simulink model "FTTest07"  (R2013a)
settings: Solver=FixedStepDiscrete  StartTime=0.0  StopTime=inf  FixedStep=0.001  RelTol=1e-3
values from neighbouring files (symbols this model uses):
  MODBUS_TIMEOUT = 0.02    [initFTTest.m]
  STREAMING_TIMEOUT = 0.1    [initFTTest.m]
undefined symbols (not defined in the file or in its folder): FTCalibration, m_XR17D15x, standard
libraries: speedgoatlib x26, xpcseriallib x13, xpclib x1, simulink x1
settings Model: BufferReuse=off  Creator=bgbuss  LastModifiedBy=bgbuss
settings DataIOCC: LimitDataPoints=off
settings OptimizationCC: BlockReduction=off  OptimizeBlockIOStorage=off  BufferReuse=off  ExpressionFolding=off  LocalBlockOutputs=off
settings DebuggingCC: UnderspecifiedInitializationDetection=Simplified
settings HardwareCC: ProdIntDivRoundTo=Zero  ProdEndianess=LittleEndian  ProdHWDeviceType=Generic->32-bit x86 compatible
settings RTWCC: SystemTargetFile=xpctarget.tlc  TemplateMakefile=xpc_default_tmf  Description=xPC Target  ProcessScript=xpctarget_make_rtw_hook  RTWCompilerOptimization=On
settings CodeAppCC: MATLABSourceComments=on
settings xpcTargetCC: TargetFcnLib=ansi_tfl_table_tmw.mat  CodeReplacementLibrary=XPC_BLAS  ParMdlRefBuildCompliant=on  ConcurrentExecutionCompliant=on  CombineSignalStateStructs=off  MATLABClassNameForMDSCustomization=xpcAperiodicCustomization  GRTInterface=on  GenerateAllocFcn=off  RL32LogBufSizeModifier=100000000  xPCTaskExecutionProfile=off  xPCRL32EventNumber=5000  xPCisModelTimeout=off  xPCModelTimeoutSecs=20  xPCLoadParamSetFile=off  xPCConcurrentTasks=off  xPCEnableSFAnimation=off

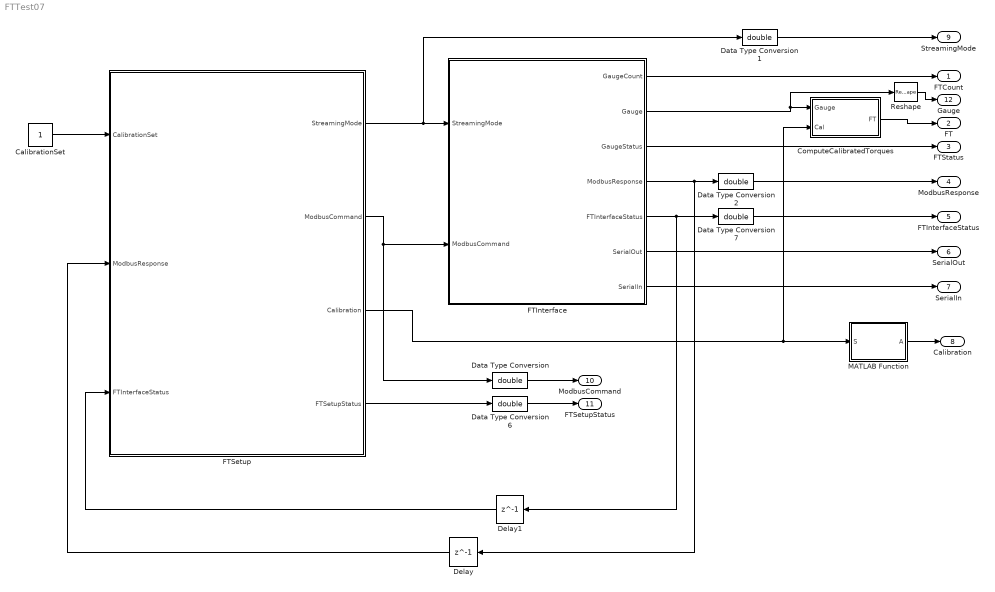
== system FTTest07 ==
  CalibrationSet : Constant
  ComputeCalibratedTorques : Subsystem
  Data Type Conversion{,1..2,6..7} (5 alike) : DataTypeConversion  OutDataTypeStr=double
  Delay : Delay  DelayLength=1  InitialCondition=zeros(256,1,'uint16')
  Delay1 : Delay  DelayLength=1  InitialCondition=0
  FTInterface : Subsystem
  FTSetup : Stateflow chart  TreatAsAtomicUnit=on
  MATLAB Function : MATLAB Function  TreatAsAtomicUnit=on
  Reshape : Reshape
  FTCount : Outport
  FT : Outport  Port=2
  FTStatus : Outport  Port=3
  ModbusResponse : Outport  Port=4
  FTInterfaceStatus : Outport  Port=5
  SerialOut : Outport  Port=6
  SerialIn : Outport  Port=7
  Calibration : Outport  Port=8
  StreamingMode : Outport  Port=9
  ModbusCommand : Outport  Port=10
  FTSetupStatus : Outport  Port=11
  Gauge : Outport  Port=12
  wires:
  FTSetup/1(StreamingMode) -> Data Type Conversion1/1, FTInterface/1(StreamingMode)
  FTInterface/1(GaugeCount) -> FTCount/1
  FTInterface/6(SerialOut) -> SerialOut/1
  FTInterface/7(SerialIn) -> SerialIn/1
  FTSetup/2(ModbusCommand) -> Data Type Conversion/1, FTInterface/2(ModbusCommand)
  FTInterface/4(ModbusResponse) -> Delay/1, Data Type Conversion2/1
  FTInterface/5(FTInterfaceStatus) -> Delay1/1, Data Type Conversion7/1
  CalibrationSet/1 -> FTSetup/1(CalibrationSet)
  FTSetup/3(Calibration) -> MATLAB Function/1(S), ComputeCalibratedTorques/2(Cal)
  MATLAB Function/1(A) -> Calibration/1
  FTInterface/2(Gauge) -> Reshape/1, ComputeCalibratedTorques/1(Gauge)
  Delay/1 -> FTSetup/2(ModbusResponse)
  Delay1/1 -> FTSetup/3(FTInterfaceStatus)
  ComputeCalibratedTorques/1(FT) -> FT/1
  Data Type Conversion/1 -> ModbusCommand/1
  Data Type Conversion1/1 -> StreamingMode/1
  Data Type Conversion2/1 -> ModbusResponse/1
  Data Type Conversion7/1 -> FTInterfaceStatus/1
  Data Type Conversion6/1 -> FTSetupStatus/1
  FTSetup/4(FTSetupStatus) -> Data Type Conversion6/1
  FTInterface/3(GaugeStatus) -> FTStatus/1
  Reshape/1 -> Gauge/1

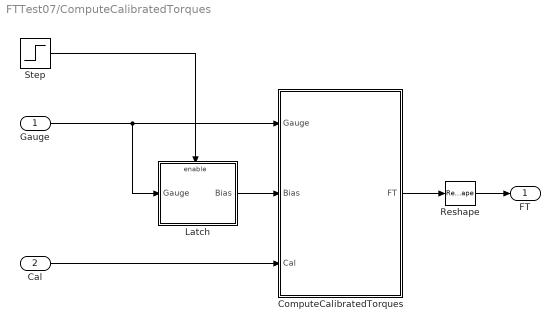
== system FTTest07/ComputeCalibratedTorques ==
  Gauge : Inport
  Cal : Inport  Port=2
  ComputeCalibratedTorques : MATLAB Function  TreatAsAtomicUnit=on
  Latch : Subsystem
  Reshape : Reshape
  Step : Step  Before=1  After=0  SampleTime=0
  FT : Outport
  wires:
  Gauge/1 -> Latch/1(Gauge), ComputeCalibratedTorques/1(Gauge)
  ComputeCalibratedTorques/1(FT) -> Reshape/1
  Cal/1 -> ComputeCalibratedTorques/3(Cal)
  Step/1 -> Latch/Enable
  Latch/1(Bias) -> ComputeCalibratedTorques/2(Bias)
  Reshape/1 -> FT/1

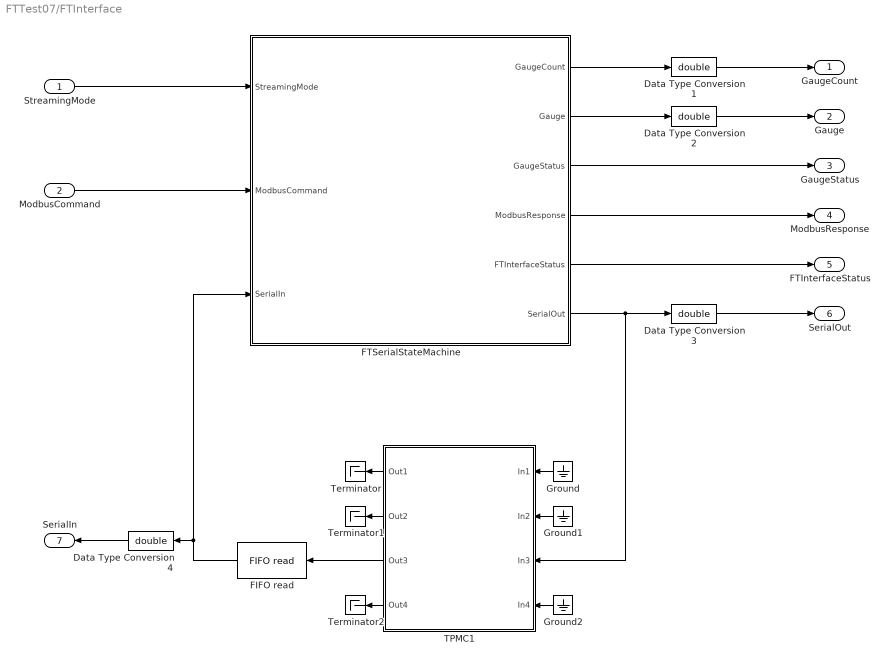
== system FTTest07/FTInterface ==
  StreamingMode : Inport
  ModbusCommand : Inport  Port=2
  Data Type Conversion{1..4} (4 alike) : DataTypeConversion  OutDataTypeStr=double
  "FIFO read " : xpcseriallib/FIFO read   maxsize=255  minsize=1  usedelimiter=off  delimiter=13  outputtype=count+16 bit uint  enable=off  enableout=off  sampletime=0.001
  FTSerialStateMachine : Stateflow chart  TreatAsAtomicUnit=on
  Ground : Ground
  Ground1 : Ground
  Ground2 : Ground
  TPMC1 : Subsystem  AncestorBlock=speedgoatlib/IO503/TPMC466  InitFcn=m_XR17D15x(3);  mask(RS232 Send Receive){group=Basic Setup, port=3, irqnum=5, slot=[4 4], transceiver1=RS485 half-duplex, standard1=on, baud1=115200, bauddivisor1=1, sampling1=16x (standard), prescale1=off, parity1=None, ndata1=8, nstop1=1, rlevel1=1, hwmode1=none, swmode1=none, xonchar1=17, xoffchar1=19, rs485auto1=off, rs485delay1=0, xmtfifosize1=1024, xmtdatatype1=8 bit uint null terminated, rcvfifosize1=1024, transceiver2=RS232 (max 921.6kb/s), standard2=on, baud2=115200, bauddivisor2=1, sampling2=16x (standard), prescale2=off, parity2=None, ndata2=8, nstop2=1, rlevel2=1, hwmode2=none, swmode2=none, xonchar2=17, xoffchar2=19, rs485auto2=off, rs485delay2=0, xmtfifosize2=1024, xmtdatatype2=8 bit uint null terminated, rcvfifosize2=1024, transceiver3=RS485 half-duplex, standard3=on, baud3=1382400, bauddivisor3=1, sampling3=16x (standard), prescale3=off, parity3=Even, ndata3=8, nstop3=1, rlevel3=1, hwmode3=none, swmode3=none, xonchar3=17, xoffchar3=19, rs485auto3=on, rs485delay3=2, xmtfifosize3=128, xmtdatatype3=count+16 bit uint, rcvfifosize3=1024, transceiver4=RS232 (max 921.6kb/s), standard4=on, baud4=115200, bauddivisor4=1, sampling4=16x (standard), prescale4=off, parity4=None, ndata4=8, nstop4=1, rlevel4=half full (32), hwmode4=none, swmode4=none, xonchar4=17, xoffchar4=19, rs485auto4=off, rs485delay4=0, xmtfifosize4=1024, xmtdatatype4=8 bit uint null terminated, rcvfifosize4=1024}
      mask prompts: group "Parameter group:"; port "Port to modify:"; irqnum "IRQ number:"; slot "PCI slot (-1: autosearch):"; transceiver1 "Transceiver setup:"; standard1 "Use standard baud rates (16x, no prescaling)"; baud1 "Standard baud rate:"; bauddivisor1 "Baud rate divisor (non-standard baud rates):"; sampling1 "Sampling rate (non-standard baud rates):"; prescale1 "Prescale by 4 (non-standard baud rates)"; parity1 "Parity:"; ndata1 "Data bits:"; nstop1 "Stop bits:"; rlevel1 "Receive FIFO interrupt level:"; hwmode1 "Hardware handshake:"; swmode1 "Software handshake:"; xonchar1 "XON character:"; xoffchar1 "XOFF character:"; rs485auto1 "RS485 auto turnaround:"; rs485delay1 "RS485 turnaround delay [0,15]"; xmtfifosize1 "Transmit software FIFO size:"; xmtdatatype1 "Transmit FIFO data type:"; rcvfifosize1 "Receive software FIFO size:"; transceiver2 "Transceiver setup:"; standard2 "Use standard baud rates (16x, no prescaling)"; baud2 "Standard baud rate:"; bauddivisor2 "Baud rate divisor (non-standard baud rates):"; sampling2 "Sampling rate (non-standard baud rates):"; prescale2 "Prescale by 4 (non-standard baud rates)"; parity2 "Parity:"; ndata2 "Data bits:"; nstop2 "Stop bits:"; rlevel2 "Receive FIFO interrupt level:"; hwmode2 "Hardware handshake:"; swmode2 "Software handshake:"; xonchar2 "XON character:"; xoffchar2 "XOFF character:"; rs485auto2 "RS485 auto turnaround:"; rs485delay2 "RS485 turnaround delay [0,15]"; xmtfifosize2 "Transmit software FIFO size:"; xmtdatatype2 "Transmit FIFO data type:"; rcvfifosize2 "Receive software FIFO size:"; transceiver3 "Transceiver setup:"; standard3 "Use standard baud rates (16x, no prescaling)"; baud3 "Standard baud rate:"; bauddivisor3 "Baud rate divisor (non-standard baud rates):"; sampling3 "Sampling rate (non-standard baud rates):"; prescale3 "Prescale by 4 (non-standard baud rates)"; parity3 "Parity:"; ndata3 "Data bits:"; nstop3 "Stop bits:"; rlevel3 "Receive FIFO interrupt level:"; hwmode3 "Hardware handshake:"; swmode3 "Software handshake:"; xonchar3 "XON character:"; xoffchar3 "XOFF character:"; rs485auto3 "RS485 auto turnaround:"; rs485delay3 "RS485 turnaround delay [0,15]"; xmtfifosize3 "Transmit software FIFO size:"; xmtdatatype3 "Transmit FIFO data type:"; rcvfifosize3 "Receive software FIFO size:"; transceiver4 "Transceiver setup:"; standard4 "Use standard baud rates (16x, no prescaling)"; baud4 "Standard baud rate:"; bauddivisor4 "Baud rate divisor (non-standard baud rates):"; sampling4 "Sampling rate (non-standard baud rates):"; prescale4 "Prescale by 4 (non-standard baud rates)"; parity4 "Parity:"; ndata4 "Data bits:"; nstop4 "Stop bits:"; rlevel4 "Receive FIFO interrupt level:"; hwmode4 "Hardware handshake:"; swmode4 "Software handshake:"; xonchar4 "XON character:"; xoffchar4 "XOFF character:"; rs485auto4 "RS485 auto turnaround:"; rs485delay4 "RS485 turnaround delay [0,15]"; xmtfifosize4 "Transmit software FIFO size:"; xmtdatatype4 "Transmit FIFO data type:"; rcvfifosize4 "Receive software FIFO size:"
      mask help:
      | PMC521
      | Acromag
      | EIA/TIA-422B Send Receive Subsystem
      mask init:
      | brdslot = slot;
      | m_tews_XR17D15x(1, 4);
      mask Help: helpview(fullfile(docroot, 'mapfiles', 'xpc.map'), 'Commtech_Subsystem')
      mask TypeOptions group: Board Setup | Basic Setup | FIFO Setup
      mask Callback group: m_tews_XR17D15x(2, 4);
      mask TypeOptions port: 1 | 2 | 3 | 4
      mask Callback port: m_tews_XR17D15x(2, 4);
      mask TypeOptions transceiver1: RS232 (max 921.6kb/s) | RS422 | RS422 multidrop | RS485 full-duplex | RS485 half-duplex
      mask TypeOptions baud1: 2764800 | 1382400 | 921600 | 460800 | 230400 | 115200 | 57600 | 38400 | 19200 | 9600 | 4800 | 2400 | 1200 | 600 | 400
      mask TypeOptions sampling1: 8x | 16x (standard)
      mask TypeOptions parity1: None | Even | Odd | Mark | Space
      mask TypeOptions ndata1: 5 | 6 | 7 | 8
      mask TypeOptions nstop1: 1 | 2
      mask TypeOptions rlevel1: 1 | quarter full (16) | half full (32) | almost full (56)
      mask TypeOptions hwmode1: RTS/CTS | none
      mask TypeOptions swmode1: XON/XOFF | none
      mask TypeOptions xmtdatatype1: count+32 bit int | count+32 bit uint | count+16 bit int | count+16 bit uint | 8 bit int null terminated | 8 bit uint null terminated
      mask TypeOptions transceiver2: RS232 (max 921.6kb/s) | RS422 | RS422 multidrop | RS485 full-duplex | RS485 half-duplex
      mask TypeOptions baud2: 2764800 | 1382400 | 921600 | 460800 | 230400 | 115200 | 57600 | 38400 | 19200 | 9600 | 4800 | 2400 | 1200 | 600 | 400
      mask TypeOptions sampling2: 8x | 16x (standard)
      mask TypeOptions parity2: None | Even | Odd | Mark | Space
      mask TypeOptions ndata2: 5 | 6 | 7 | 8
      mask TypeOptions nstop2: 1 | 2
      mask TypeOptions rlevel2: 1 | quarter full (16) | half full (32) | almost full (56)
      mask TypeOptions hwmode2: RTS/CTS | none
      mask TypeOptions swmode2: XON/XOFF | none
      mask TypeOptions xmtdatatype2: count+32 bit int | count+32 bit uint | count+16 bit int | count+16 bit uint | 8 bit int null terminated | 8 bit uint null terminated
      mask TypeOptions transceiver3: RS232 (max 921.6kb/s) | RS422 | RS422 multidrop | RS485 full-duplex | RS485 half-duplex
      mask TypeOptions baud3: 2764800 | 1382400 | 921600 | 460800 | 230400 | 115200 | 57600 | 38400 | 19200 | 9600 | 4800 | 2400 | 1200 | 600 | 400
      mask TypeOptions sampling3: 8x | 16x (standard)
      mask TypeOptions parity3: None | Even | Odd | Mark | Space
      mask TypeOptions ndata3: 5 | 6 | 7 | 8
      mask TypeOptions nstop3: 1 | 2
      mask TypeOptions rlevel3: 1 | quarter full (16) | half full (32) | almost full (56)
      mask TypeOptions hwmode3: RTS/CTS | none
      mask TypeOptions swmode3: XON/XOFF | none
      mask TypeOptions xmtdatatype3: count+32 bit int | count+32 bit uint | count+16 bit int | count+16 bit uint | 8 bit int null terminated | 8 bit uint null terminated
      mask TypeOptions transceiver4: RS232 (max 921.6kb/s) | RS422 | RS422 multidrop | RS485 full-duplex | RS485 half-duplex
      mask TypeOptions baud4: 2764800 | 1382400 | 921600 | 460800 | 230400 | 115200 | 57600 | 38400 | 19200 | 9600 | 4800 | 2400 | 1200 | 600 | 400
      mask TypeOptions sampling4: 8x | 16x (standard)
      mask TypeOptions parity4: None | Even | Odd | Mark | Space
      mask TypeOptions ndata4: 5 | 6 | 7 | 8
      mask TypeOptions nstop4: 1 | 2
      mask TypeOptions rlevel4: 1 | quarter full (16) | half full (32) | almost full (56)
      mask TypeOptions hwmode4: RTS/CTS | none
      mask TypeOptions swmode4: XON/XOFF | none
      mask TypeOptions xmtdatatype4: count+32 bit int | count+32 bit uint | count+16 bit int | count+16 bit uint | 8 bit int null terminated | 8 bit uint null terminated
      mask Display:
      | disp('TEWS\nTPMC466\nRS232/422/485\nSend\nReceive');
      | port_label( 'input', 1, 'XMT1' );
      | port_label( 'input', 2, 'XMT2' );
      | port_label( 'input', 3, 'XMT3' );
      | port_label( 'input', 4, 'XMT4' );
      | 
      | port_label( 'output', 1, 'FIFO1' );
      | port_label( 'output', 2, 'FIFO2' );
      | port_label( 'output', 3, 'FIFO3' );
      | port_label( 'output', 4, 'FIFO4' );
  Terminator : Terminator
  Terminator1 : Terminator
  Terminator2 : Terminator
  GaugeCount : Outport
  Gauge : Outport  Port=2
  GaugeStatus : Outport  Port=3
  ModbusResponse : Outport  Port=4
  FTInterfaceStatus : Outport  Port=5
  SerialOut : Outport  Port=6
  SerialIn : Outport  Port=7
  wires:
  FTSerialStateMachine/2(Gauge) -> Data Type Conversion2/1
  Data Type Conversion2/1 -> Gauge/1
  FTSerialStateMachine/1(GaugeCount) -> Data Type Conversion1/1
  TPMC1/3(Out3) -> "FIFO read "/1
  ModbusCommand/1 -> FTSerialStateMachine/2(ModbusCommand)
  TPMC1/1(Out1) -> Terminator/1
  TPMC1/2(Out2) -> Terminator1/1
  TPMC1/4(Out4) -> Terminator2/1
  Ground/1 -> TPMC1/1(In1)
  Ground2/1 -> TPMC1/4(In4)
  Ground1/1 -> TPMC1/2(In2)
  FTSerialStateMachine/4(ModbusResponse) -> ModbusResponse/1
  Data Type Conversion1/1 -> GaugeCount/1
  Data Type Conversion3/1 -> SerialOut/1
  "FIFO read "/1 -> Data Type Conversion4/1, FTSerialStateMachine/3(SerialIn)
  Data Type Conversion4/1 -> SerialIn/1
  StreamingMode/1 -> FTSerialStateMachine/1(StreamingMode)
  FTSerialStateMachine/5(FTInterfaceStatus) -> FTInterfaceStatus/1
  FTSerialStateMachine/6(SerialOut) -> Data Type Conversion3/1, TPMC1/3(In3)
  FTSerialStateMachine/3(GaugeStatus) -> GaugeStatus/1

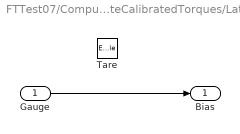
== system FTTest07/ComputeCalibratedTorques/Latch ==
  Gauge : Inport
  Tare : EnablePort
  Bias : Outport  InitialOutput=zeros(6,8,'uint16')
  wires:
  Gauge/1 -> Bias/1

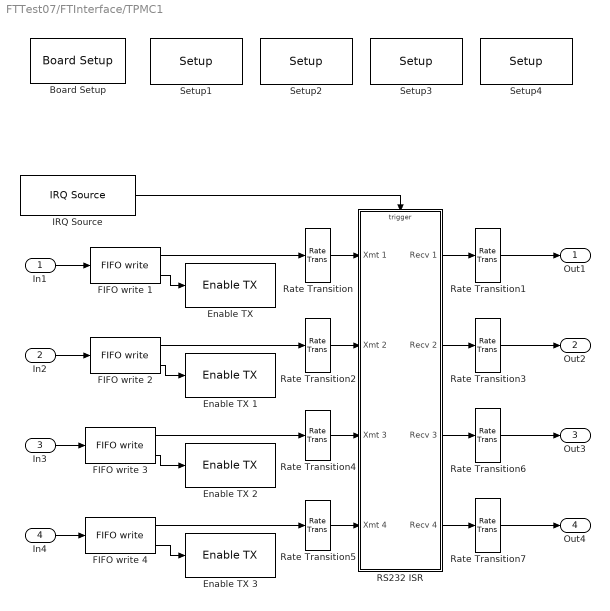
== system FTTest07/FTInterface/TPMC1 ==
  In1 : Inport
  In2 : Inport  Port=2
  In3 : Inport  Port=3
  In4 : Inport  Port=4
  Board Setup : speedgoatlib/IO503/TEWS TPMC466 Internal blocks/Board Setup  irqnum=5  slot=brdslot
  "Enable TX " : speedgoatlib/IO503/TEWS TPMC466 Internal blocks/Enable TX   port=1  slot=brdslot
  Enable TX 1 : speedgoatlib/IO503/TEWS TPMC466 Internal blocks/Enable TX   port=2  slot=brdslot
  Enable TX 2 : speedgoatlib/IO503/TEWS TPMC466 Internal blocks/Enable TX   port=3  slot=brdslot
  Enable TX 3 : speedgoatlib/IO503/TEWS TPMC466 Internal blocks/Enable TX   port=4  slot=brdslot
  FIFO write 1 : xpcseriallib/FIFO write   size=1024  inputtype=8 bit uint null terminated  present=on  sampletime=-1  id=XMT channel 1, IRQ 5
  FIFO write 2 : xpcseriallib/FIFO write   size=1024  inputtype=8 bit uint null terminated  present=on  sampletime=-1  id=XMT channel 2, IRQ 5
  FIFO write 3 : xpcseriallib/FIFO write   size=128  inputtype=count+16 bit uint  present=on  sampletime=-1  id=XMT channel 3, IRQ 5
  FIFO write 4 : xpcseriallib/FIFO write   size=1024  inputtype=8 bit uint null terminated  present=on  sampletime=-1  id=XMT channel 4, IRQ 5
  IRQ Source : xpclib/Asynchronous Event/IRQ Source  irqNo=5  preempt=off  b_type=None/Other  slot=brdslot
  RS232 ISR : Subsystem  TreatAsAtomicUnit=on  mask(RS232 ISR){slot=brdslot}
      mask help:
      | PMC521
      | Acromag
      | Interrupt Service Routine
      mask init:
      | subslot = slot;
      mask Display:
      | disp('PMC521\nAcromag\nISR');
      | port_label('input', 1, 'XMT1');
      | port_label('input', 2, 'XMT2');
      | port_label('input', 3, 'XMT3');
      | port_label('input', 4, 'XMT4');
      | port_label('input', 5, 'XMT5');
      | port_label('input', 6, 'XMT6');
      | port_label('input', 7, 'XMT7');
      | port_label('input', 8, 'XMT8');
      | port_label('output', 1, 'RCV1');
      | port_label('output', 2, 'RCV2');
      | port_label('output', 3, 'RCV3');
      | port_label('output', 4, 'RCV4');
      | port_label('output', 5, 'RCV5');
      | port_label('output', 6, 'RCV6');
      | port_label('output', 7, 'RCV7');
      | port_label('output', 8, 'RCV8');
  Rate Transition{,2,4..5} (4 alike) : RateTransition  Integrity=off  Deterministic=off
  Rate Transition{1,3,6..7} (4 alike) : RateTransition  Integrity=off  Deterministic=off  OutPortSampleTime=0
  Setup1 : speedgoatlib/IO503/TEWS TPMC466 Internal blocks/Setup   port=1  transceiver=RS485 half-duplex  standard=on  baudrate=115200  bauddivisor=1  mode8x=16x (standard)  prescale=off  width=8  nstop=1  parity=None  rlevel=1  ctsmode=none  xonoff=none  xon=17  xoff=19  rs485mode=off  rs485delay=0  slot=brdslot
  Setup2 : speedgoatlib/IO503/TEWS TPMC466 Internal blocks/Setup   port=2  transceiver=RS232 (max 921.6kb/s)  standard=on  baudrate=115200  bauddivisor=1  mode8x=16x (standard)  prescale=off  width=8  nstop=1  parity=None  rlevel=1  ctsmode=none  xonoff=none  xon=17  xoff=19  rs485mode=off  rs485delay=0  slot=brdslot
  Setup3 : speedgoatlib/IO503/TEWS TPMC466 Internal blocks/Setup   port=3  transceiver=RS485 half-duplex  standard=on  baudrate=1382400  bauddivisor=1  mode8x=16x (standard)  prescale=off  width=8  nstop=1  parity=Even  rlevel=1  ctsmode=none  xonoff=none  xon=17  xoff=19  rs485mode=on  rs485delay=2  slot=brdslot
  Setup4 : speedgoatlib/IO503/TEWS TPMC466 Internal blocks/Setup   port=4  transceiver=RS232 (max 921.6kb/s)  standard=on  baudrate=115200  bauddivisor=1  mode8x=16x (standard)  prescale=off  width=8  nstop=1  parity=None  rlevel=half full (32)  ctsmode=none  xonoff=none  xon=17  xoff=19  rs485mode=off  rs485delay=0  slot=brdslot
  Out1 : Outport
  Out2 : Outport  Port=2
  Out3 : Outport  Port=3
  Out4 : Outport  Port=4
  wires:
  RS232 ISR/4(Recv 4) -> Rate Transition7/1
  RS232 ISR/3(Recv 3) -> Rate Transition6/1
  Rate Transition7/1 -> Out4/1
  Rate Transition6/1 -> Out3/1
  Rate Transition5/1 -> RS232 ISR/4(Xmt 4)
  Rate Transition4/1 -> RS232 ISR/3(Xmt 3)
  FIFO write 4/1 -> Rate Transition5/1
  In4/1 -> FIFO write 4/1
  FIFO write 4/2 -> Enable TX 3/1
  FIFO write 3/1 -> Rate Transition4/1
  In3/1 -> FIFO write 3/1
  FIFO write 3/2 -> Enable TX 2/1
  Rate Transition1/1 -> Out1/1
  Rate Transition3/1 -> Out2/1
  Rate Transition/1 -> RS232 ISR/1(Xmt 1)
  Rate Transition2/1 -> RS232 ISR/2(Xmt 2)
  FIFO write 1/2 -> "Enable TX "/1
  IRQ Source/1 -> RS232 ISR/Trigger
  RS232 ISR/1(Recv 1) -> Rate Transition1/1
  RS232 ISR/2(Recv 2) -> Rate Transition3/1
  FIFO write 1/1 -> Rate Transition/1
  In1/1 -> FIFO write 1/1
  FIFO write 2/1 -> Rate Transition2/1
  In2/1 -> FIFO write 2/1
  FIFO write 2/2 -> Enable TX 1/1

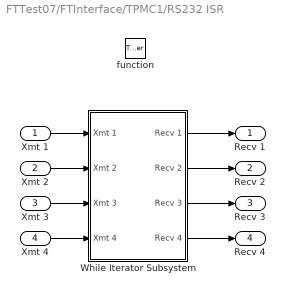
== system FTTest07/FTInterface/TPMC1/RS232 ISR ==
  Xmt 1 : Inport
  Xmt 2 : Inport  Port=2
  Xmt 3 : Inport  Port=3
  Xmt 4 : Inport  Port=4
  function : TriggerPort  TriggerType=function-call
  While Iterator Subsystem : Subsystem  TreatAsAtomicUnit=on
  Recv 1 : Outport  SourceOfInitialOutputValue=Input signal
  Recv 2 : Outport  Port=2  SourceOfInitialOutputValue=Input signal
  Recv 3 : Outport  Port=3  SourceOfInitialOutputValue=Input signal
  Recv 4 : Outport  Port=4  SourceOfInitialOutputValue=Input signal
  wires:
  While Iterator Subsystem/4(Recv 4) -> Recv 4/1
  While Iterator Subsystem/3(Recv 3) -> Recv 3/1
  Xmt 4/1 -> While Iterator Subsystem/4(Xmt 4)
  Xmt 3/1 -> While Iterator Subsystem/3(Xmt 3)
  While Iterator Subsystem/2(Recv 2) -> Recv 2/1
  While Iterator Subsystem/1(Recv 1) -> Recv 1/1
  Xmt 2/1 -> While Iterator Subsystem/2(Xmt 2)
  Xmt 1/1 -> While Iterator Subsystem/1(Xmt 1)

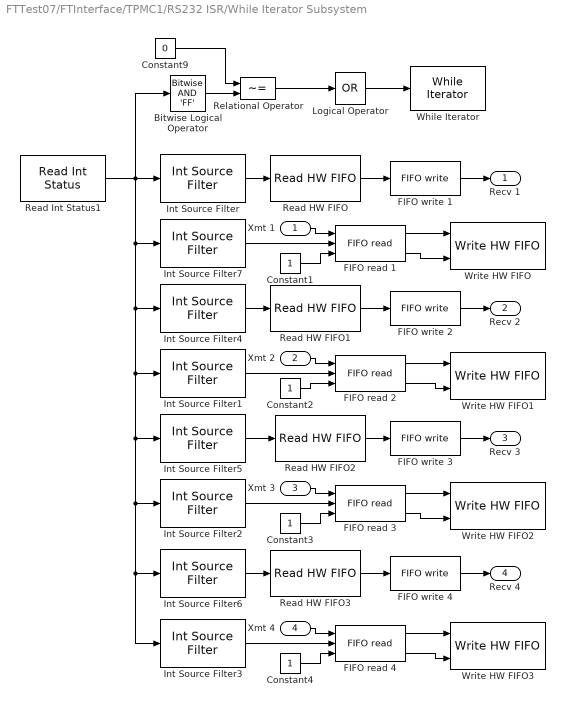
== system FTTest07/FTInterface/TPMC1/RS232 ISR/While Iterator Subsystem ==
  Xmt 1 : Inport
  Xmt 2 : Inport  Port=2
  Xmt 3 : Inport  Port=3
  Xmt 4 : Inport  Port=4
  Bitwise Logical Operator : simulink/Logic and Bit Operations/Bitwise Operator  logicop=AND  UseBitMask=on  BitMask='FF'  BitMaskRealWorld=Stored Integer
  Constant{1..4} (4 alike) : Constant  OutDataTypeStr=uint32
  Constant9 : Constant  Value=0  OutDataTypeStr=uint32
  FIFO read {1..4} (4 alike) : xpcseriallib/FIFO read   maxsize=60  minsize=1  usedelimiter=off  delimiter=13  outputtype=count+32 bit uint  enable=on  enableout=on  sampletime=-1
  FIFO write 1 : xpcseriallib/FIFO write   size=1024  inputtype=count+32 bit uint  present=off  sampletime=-1  id=RCV channel 1, IRQ 5
  FIFO write 2 : xpcseriallib/FIFO write   size=1024  inputtype=count+32 bit uint  present=off  sampletime=-1  id=RCV channel 2, IRQ 5
  FIFO write 3 : xpcseriallib/FIFO write   size=1024  inputtype=count+32 bit uint  present=off  sampletime=-1  id=RCV channel 3, IRQ 5
  FIFO write 4 : xpcseriallib/FIFO write   size=1024  inputtype=count+32 bit uint  present=off  sampletime=-1  id=RCV channel 4, IRQ 5
  Int Source Filter : speedgoatlib/IO503/TEWS TPMC466 Internal blocks/Int Source Filter  port=1  value=Receive data
  Int Source Filter1 : speedgoatlib/IO503/TEWS TPMC466 Internal blocks/Int Source Filter  port=2  value=Transmitter empty
  Int Source Filter2 : speedgoatlib/IO503/TEWS TPMC466 Internal blocks/Int Source Filter  port=3  value=Transmitter empty
  Int Source Filter3 : speedgoatlib/IO503/TEWS TPMC466 Internal blocks/Int Source Filter  port=4  value=Transmitter empty
  Int Source Filter4 : speedgoatlib/IO503/TEWS TPMC466 Internal blocks/Int Source Filter  port=2  value=Receive data
  Int Source Filter5 : speedgoatlib/IO503/TEWS TPMC466 Internal blocks/Int Source Filter  port=3  value=Receive data
  Int Source Filter6 : speedgoatlib/IO503/TEWS TPMC466 Internal blocks/Int Source Filter  port=4  value=Receive data
  Int Source Filter7 : speedgoatlib/IO503/TEWS TPMC466 Internal blocks/Int Source Filter  port=1  value=Transmitter empty
  Logical Operator : Logic  Operator=OR  Inputs=1  AllPortsSameDT=off
  Read HW FIFO : speedgoatlib/IO503/TEWS TPMC466 Internal blocks/Read HW FIFO  port=1  flush=on  slot=subslot
  Read HW FIFO1 : speedgoatlib/IO503/TEWS TPMC466 Internal blocks/Read HW FIFO  port=2  flush=on  slot=subslot
  Read HW FIFO2 : speedgoatlib/IO503/TEWS TPMC466 Internal blocks/Read HW FIFO  port=3  flush=on  slot=subslot
  Read HW FIFO3 : speedgoatlib/IO503/TEWS TPMC466 Internal blocks/Read HW FIFO  port=4  flush=on  slot=subslot
  Read Int Status1 : speedgoatlib/IO503/TEWS TPMC466 Internal blocks/Read Int Status  slot=subslot
  Relational Operator : RelationalOperator  Operator=~=
  While Iterator : WhileIterator  MaxIters=65  WhileBlockType=do-while
  Write HW FIFO : speedgoatlib/IO503/TEWS TPMC466 Internal blocks/Write HW FIFO  port=1  slot=subslot
  Write HW FIFO1 : speedgoatlib/IO503/TEWS TPMC466 Internal blocks/Write HW FIFO  port=2  slot=subslot
  Write HW FIFO2 : speedgoatlib/IO503/TEWS TPMC466 Internal blocks/Write HW FIFO  port=3  slot=subslot
  Write HW FIFO3 : speedgoatlib/IO503/TEWS TPMC466 Internal blocks/Write HW FIFO  port=4  slot=subslot
  Recv 1 : Outport  SourceOfInitialOutputValue=Input signal
  Recv 2 : Outport  Port=2  SourceOfInitialOutputValue=Input signal
  Recv 3 : Outport  Port=3  SourceOfInitialOutputValue=Input signal
  Recv 4 : Outport  Port=4  SourceOfInitialOutputValue=Input signal
  wires:
  Read HW FIFO3/1 -> FIFO write 4/1
  FIFO write 4/1 -> Recv 4/1
  Read HW FIFO2/1 -> FIFO write 3/1
  FIFO write 3/1 -> Recv 3/1
  Int Source Filter6/1 -> Read HW FIFO3/1
  Int Source Filter5/1 -> Read HW FIFO2/1
  Constant3/1 -> FIFO read 3/3
  FIFO read 3/2 -> Write HW FIFO2/2
  FIFO read 3/1 -> Write HW FIFO2/1
  Xmt 3/1 -> FIFO read 3/1
  Int Source Filter2/1 -> FIFO read 3/2
  Constant2/1 -> FIFO read 2/3
  Constant1/1 -> FIFO read 1/3
  FIFO read 2/2 -> Write HW FIFO1/2
  FIFO read 1/2 -> Write HW FIFO/2
  FIFO read 1/1 -> Write HW FIFO/1
  FIFO read 2/1 -> Write HW FIFO1/1
  Xmt 2/1 -> FIFO read 2/1
  Int Source Filter1/1 -> FIFO read 2/2
  Read HW FIFO1/1 -> FIFO write 2/1
  FIFO write 2/1 -> Recv 2/1
  Int Source Filter4/1 -> Read HW FIFO1/1
  Xmt 1/1 -> FIFO read 1/1
  Int Source Filter7/1 -> FIFO read 1/2
  Read HW FIFO/1 -> FIFO write 1/1
  FIFO write 1/1 -> Recv 1/1
  Int Source Filter/1 -> Read HW FIFO/1
  Read Int Status1/1 -> Bitwise Logical Operator/1, Int Source Filter6/1, Int Source Filter3/1, Int Source Filter2/1, Int Source Filter5/1, Int Source Filter1/1, Int Source Filter4/1, Int Source Filter7/1, Int Source Filter/1
  Constant9/1 -> Relational Operator/1
  Bitwise Logical Operator/1 -> Relational Operator/2
  Relational Operator/1 -> Logical Operator/1
  Logical Operator/1 -> While Iterator/1
  Constant4/1 -> FIFO read 4/3
  FIFO read 4/2 -> Write HW FIFO3/2
  FIFO read 4/1 -> Write HW FIFO3/1
  Xmt 4/1 -> FIFO read 4/1
  Int Source Filter3/1 -> FIFO read 4/2

== stateflow chart FTTest07/FTSetup ==
  state Initialize
    entry:
    FTSetupStatus = 0;
    clearModbusCommand();
    clearCalibration();
    StreamingMode = 0;
  state ModbusMode
    entry:
    FTSetupStatus = 1;
    clearModbusCommand();
    clearCalibration();
    StreamingMode = 0;
    state SetSessionId
      entry:
      FTSetupStatus = 1.10;
    state ReadCalibration
      entry:
      FTSetupStatus = 1.20;
      state SendRequest1
        entry:
        FTSetupStatus = 1.21;
        requestCalibration(1);
        during:
        clearModbusCommand();
      state SendRequest2
        entry:
        FTSetupStatus = 1.23;
        requestCalibration(2);
        during:
        clearModbusCommand();
      state ParseRequest1
        entry:
        FTSetupStatus = 1.22;
        parseCalibration(1);
      state ParseRequest2
        entry:
        FTSetupStatus = 1.24;
        parseCalibration(2);
      (default) -> SendRequest1
      SendRequest1 -> SendRequest1 [order 2] : [after(0.2,sec)]
      SendRequest2 -> SendRequest2 [order 2] : [after(0.2, sec)]
      ParseRequest1 -> SendRequest2
      SendRequest1 -> ParseRequest1 [order 1] : [validResponse()]
      SendRequest2 -> ParseRequest2 [order 1] : [validResponse()]
    state WriteActiveCalibration
      entry:
      FTSetupStatus = 1.30;
      (history)
      state LockStorage
        entry:
        FTSetupStatus = 1.34;
        lockUnlockStorage(0);
        during:
        clearModbusCommand();
      state writeActiveCal
        entry:
        FTSetupStatus = 1.33;
        writeActiveCalibration();
        during:
        clearModbusCommand();
      state readActiveCal
        entry:
        FTSetupStatus = 1.31;
        readActiveCalibration();
        during:
        clearModbusCommand();
      state UnlockStorage
        entry:
        FTSetupStatus = 1.32;
        lockUnlockStorage(1);
        during:
        clearModbusCommand();
      (default) -> readActiveCal
      writeActiveCal -> LockStorage : [validResponse()]
      LockStorage -> readActiveCal : [validResponse()]
      UnlockStorage -> writeActiveCal : [validResponse()]
      readActiveCal -> UnlockStorage [order 2] : [validResponse()]
    (default) -> SetSessionId
    SetSessionId -> ReadCalibration
    ParseRequest2 -> WriteActiveCalibration
    WriteActiveCalibration -> WriteActiveCalibration : [after(2*MODBUS_TIMEOUT, sec)]
  state StreamingMode
    entry:
    FTSetupStatus = 2;
    clearModbusCommand();
    StreamingMode = 1;
  (default) -> Initialize
  Initialize -> ModbusMode : [abs(FTInterfaceStatus - 1.1) < 0.0001]
  readActiveCal -> StreamingMode [order 1] : [validResponse() && verifyActiveCalibration()]
  data: valid function_output; Part function_input; Part function_input; ok function_output; Unlock function_input; CalibrationSet input; StreamingMode output; ModbusResponse input; FTInterfaceStatus input; ModbusCommand output uint16 size=256; Calibration output Bus: FTCalibrationBus; FTCalibration parameter Bus: FTCalibrationBus; FTSetupStatus output; CalibrationBuffer local; CalibrationBufferEnd local; MODBUS_TIMEOUT parameter
  function clearModbusCommand:
    | function clearModbusCommand %#codegen
    |     ModbusCommand = zeros(256,1,'uint16');
    | end
  function clearCalibration:
    | function clearCalibration %#codegen
    |     Calibration       = FTCalibration;
    |     CalibrationBuffer = zeros(512,1,'uint16');
    |     CalibrationBufferEnd = uint16(0);
    | end
  function valid = validResponse:
    | function valid = validResponse %#codegen
    |     valid = false;
    |     
    |     if (ModbusResponse(1) > 1)    
    |         switch (ModbusResponse(2))
    |             case uint16(3)
    |                 valid = true;
    |             case uint16(6)
    |                 valid = true;
    |             case uint16(16)
    |                 valid = true;
    |             case uint16(70)
    |                 valid = (ModbusResponse(3) == uint16(1));
    |             case uint16(106)
    |                 valid = (ModbusResponse(3) == uint16(1));
    |         end
    |     end
    | end
  function requestCalibration(Part):
    | function requestCalibration(Part) %#codegen
    |    % ATI F/T Calibration data are stored in holding registers. There are 16
    |    % calibration sets, each 338 bytes (or 169 16-bit holding registers)
    |    % long. They are stored beginning at holding register address 0x00e3
    |    % (Calibration 1) 192 holding registers apart.
    |    Address = uint16(hex2dec('00e3')) + uint16(192 * (CalibrationSet - 1));
    |    
    |    % Calibration data must be read in two or more parts due to length
    |    % restricitons in the Modbus protocol.
    |    NumRegs1 = 85;
    |    NumRegs2 = 84;
    |    if (Part==1)
    |        NumRegs = NumRegs1;
    |    else
    |        NumRegs = NumRegs2;
    |        Address = Address + uint16(NumRegs1);
    |    end
    |    ModbusFunction = 3;
    |    ModbusCommand(1:6) = uint16([5; ModbusFunction; bitshift(Address,-8); bitand(Address,255); 0; NumRegs]);
    | end
  function parseCalibration(Part):
    | function parseCalibration(Part) %#codegen
    |     % Calibration data must be read in two or more parts due to length
    |     % restricitons in the Modbus protocol.
    |     if (Part==1)
    |         CalibrationBuffer(1:ModbusResponse(3)) = ModbusResponse(3+(1:ModbusResponse(3)));
    |         CalibrationBufferEnd = ModbusResponse(3);
    |     else
    |         CalibrationBuffer(CalibrationBufferEnd+(1:ModbusResponse(3))) = ModbusResponse(3+(1:ModbusResponse(3)));
    |         CalibrationBufferEndTemp = CalibrationBufferEnd + ModbusResponse(3);
    |         Calibration = parseFTCalibration2(CalibrationBuffer(1:CalibrationBufferEndTemp));
    |     end
    | end
    | 
    | function Cal = parseFTCalibration2(CalibrationBuffer)
    |     Cal.CalibSerialNumber = parseUint8(CalibrationBuffer(1:8));
    |     Cal.CalibPartNumber   = parseUint8(CalibrationBuffer(9:40));
    |     Cal.CalibFamilyId     = parseUint8(CalibrationBuffer(41:44));
    |     Cal.CalibTime         = parseUint8(CalibrationBuffer(45:64));
    |     Cal.BasicMatrix       = reshape(parseFloat(CalibrationBuffer(65:208)), 6, 6).';
    |     Cal.ForceUnits        = parseUint8(CalibrationBuffer(209));
    |     Cal.TorqueUnits       = parseUint8(CalibrationBuffer(210));
    |     Cal.MaxRating         = parseFloat(CalibrationBuffer(211:234));
    |     Cal.CountsPerForce    = parseInt32(CalibrationBuffer(235:238));
    |     Cal.CountsPerTorque   = parseInt32(CalibrationBuffer(239:242));
    |     Cal.GageGain          = parseUint16(CalibrationBuffer(243:254));
    |     Cal.GageOffset        = parseUint16(CalibrationBuffer(255:266));
    |     Cal.Resolution        = parseUint8(CalibrationBuffer(267:272));
    |     Cal.Range             = parseUint8(CalibrationBuffer(273:278));
    |     Cal.ScaleFactor16     = parseUint16(CalibrationBuffer(279:290));
    |     Cal.UserField1        = parseUint8(CalibrationBuffer(291:306));
    |     Cal.UserField2        = parseUint8(CalibrationBuffer(307:322));
    |     Cal.SpareData         = parseUint8(CalibrationBuffer(323:338));
    | end
    | 
    | 
    | function d = parseUint8(D)
    |     d = double(D);
    | end
    | 
    | function d = parseFloat(D)
    |     D1 = uint32(D);
    |     D2 = bitshift(D1(1:4:end), 24) + bitshift(D1(2:4:end), 16) + bitshift(D1(3:4:end), 8) + D1(4:4:end);
    |     d = double(typecast(D2, 'single'));
    | end
    | 
    | function d = parseUint32(D)
    |     D1 = uint32(D);
    |     D2 = bitshift(D1(1:4:end), 24) + bitshift(D1(2:4:end), 16) + bitshift(D1(3:4:end), 8) + D1(4:4:end);
    |     d  = double(D2);
    | end
    | 
    | function d = parseInt32(D)
    |     D1 = int32(D);
    |     D2 = bitshift(D1(1:4:end), 24) + bitshift(D1(2:4:end), 16) + bitshift(D1(3:4:end), 8) + D1(4:4:end);
    |     d  = double(D2);
    | end
    | 
    | function d = parseUint16(D)
    |     D1 = uint16(D);
    |     D2 = bitshift(D1(1:2:end), 8) + D1(2:2:end);
    |     d  = double(D2);
    | end
  function writeActiveCalibration:
    | function writeActiveCalibration %#codegen
    |     % ATI F/T Calibration data are stored in holding registers. After
    |     % reading a calibration data set, we must write the GaugeGain and
    |     % GaugeOffset values to the active gain and offset holding registers.
    |     % Holding register addresses:
    |     %   0x0000-0x0005 Active Gain pots
    |     %   0x0006-0x000B Active Offset DACs
    |     ModbusFunction = 16; % Write multiple registers
    |     Address = uint16(0);
    |     NumRegs = 12;
    |     
    |     ModbusCommand(1:31) = uint16([30; ModbusFunction; bitshift(Address,-8); bitand(Address,255); 0; NumRegs; 2*NumRegs; zeros(2*NumRegs,1, 'uint16')]);
    |     
    |     Data = uint16([Calibration.GageGain Calibration.GageOffset]);
    |     for k=1:NumRegs
    |         ModbusCommand(8 + 2*(k-1)) = bitshift(Data(k), -8); 
    |         ModbusCommand(9 + 2*(k-1)) = bitand(Data(k), 255);
    |     end
    | end
  function ok = verifyActiveCalibration:
    | function ok = verifyActiveCalibration %#codegen
    |     % ATI F/T Calibration data are stored in holding registers. After
    |     % reading a calibration data set, we must write the GaugeGain and
    |     % GaugeOffset values to the active gain and offset holding registers.
    |     % Holding register addresses:
    |     %   0x0000-0x0005 Active Gain pots
    |     %   0x0006-0x000B Active Offset DACs
    |     ok = false;
    |     
    |     % Check response length
    |     if (ModbusResponse(1) ~= uint16(26))
    |         return
    |     end
    |     
    |     % Compare gain and offset values with those in the calibration
    |     % structure
    |     ActiveGaugeGain   = parseUint16(ModbusResponse(3  + (1:12)));
    |     ActiveGaugeOffset = parseUint16(ModbusResponse(15 + (1:12)));
    |     
    |     if any(ActiveGaugeGain ~= Calibration.GageGain) ...
    |             || any(ActiveGaugeOffset ~= Calibration.GageOffset)
    |         return;
    |     end
    |     
    |     % Then it looks okay
    |     ok = true;
    | end
    | 
    | function u = parseUint16(D)
    |     D1 = double(D);
    |     u = D1(1:2:end)*256 + D1(2:2:end);
    | end
  function lockUnlockStorage(Unlock):
    | function lockUnlockStorage(Unlock) %#codegen
    |     % ATI F/T Calibration data are stored in holding registers. After
    |     % reading a calibration data set, we must write the GaugeGain and
    |     % GaugeOffset values to the active gain and offset holding registers.
    |     % Before writing to the active gain/offset registers, we must unlock
    |     % the storage.
    |     
    |     ModbusFunction = 106; % Read holding registers
    |     if (Unlock==1)
    |         Data = 170; % hex2dec('aa')
    |     else
    |         Data = 24; % hex2dec('18')
    |     end
    |         
    |     ModbusCommand(1:3) = uint16([2; ModbusFunction; Data]);
    | end
  function readActiveCalibration:
    | function readActiveCalibration %#codegen
    |     % ATI F/T Calibration data are stored in holding registers. After
    |     % reading a calibration data set, we must write the GaugeGain and
    |     % GaugeOffset values to the active gain and offset holding registers.
    |     % Holding register addresses:
    |     %   0x0000-0x0005 Active Gain pots
    |     %   0x0006-0x000B Active Offset DACs
    |     ModbusFunction = 3; % Read holding registers
    |     Address = uint16(0);
    |     NumRegs = 12;
    |     ModbusCommand(1:6) = uint16([5; ModbusFunction; bitshift(Address,-8); bitand(Address,255); 0; NumRegs]);
    | end

== matlab function FTTest07/MATLAB Function ==
  data: S input; A output
function A = fcn(S)
    %#codegen
    A = serializeFTCalibrationBus(S);
end

== stateflow chart FTTest07/FTInterface/FTSerialStateMachine ==
  state StreamingMode
    entry:
    FTInterfaceStatus = 2;
    clearGauge();
    clearSerialOut();
    clearSerialBuffer();
    during:
    parseStreamingData();
  state ModbusMode
    entry:
    FTInterfaceStatus = 1;
    clearGauge();
    clearSerialOut();
    state ModbusIdle
      entry:
      FTInterfaceStatus = 1.1;
      clearModbusResponse();
      clearSerialBuffer();
    state ModbusSend
      entry:
      FTInterfaceStatus = 1.2;
      clearSerialBuffer();
      sendModbusCmd(ModbusCommand);
      exit:
      clearSerialOut();
    state ModbusReceive
      entry, during:
      FTInterfaceStatus = 1.3;
      readModbusResponse()
    state ModbusValidate
      entry:
      FTInterfaceStatus = 1.4;
      validateModbusResponse();
      exit:
      clearModbusResponse();
    (default) -> ModbusIdle
    (junction 37) -> ModbusIdle
    (junction 99) -> (junction 37) [order 2]
    ModbusIdle -> ModbusSend [order 2] : [ModbusCommand(1)>0]
    (junction 99) -> ModbusSend [order 1] : [ModbusCommand(1)>0]
    (junction 36) -> (junction 99)
    ModbusSend -> ModbusReceive
    ModbusReceive -> (junction 36) [order 2] : [after(MODBUS_TIMEOUT, sec)]
    (junction 86) -> (junction 36)
    ModbusReceive -> ModbusValidate [order 1] : [Valid]
    ModbusValidate -> (junction 86)
  state InitializeStreaming
    entry:
    FTInterfaceStatus = 3;
    clearSerialBuffer();
    sendStreamingCmd(1);
    exit:
    clearSerialOut();
  state CheckStreaming
    state WaitClear
      entry:
      FTInterfaceStatus = 0.1;
      clearSerialOut();
      clearSerialBuffer();
    state CheckSerialInput
      entry:
      FTInterfaceStatus = 0.2;
    (default) -> WaitClear
    WaitClear -> CheckSerialInput
  state EndStreaming
    entry:
    FTInterfaceStatus = 4;
    clearSerialBuffer();
    sendStreamingCmd(0);
    exit:
    clearSerialOut();
  ModbusIdle -> InitializeStreaming [order 1] : [StreamingMode~=0]
  InitializeStreaming -> CheckStreaming
  (default) -> CheckStreaming
  CheckSerialInput -> ModbusMode [order 2] : [after(STREAMING_TIMEOUT, sec)]
  CheckSerialInput -> StreamingMode [order 1] : [SerialIn(1)>0]
  EndStreaming -> CheckStreaming
  StreamingMode -> EndStreaming : [StreamingMode==0]
  data: Command function_input; Select function_input; StreamingMode input; SerialBuffer local; SerialBufferEnd local; GaugeCount output; Gauge output size=[6 8]; GaugeStatus output; ModbusCommand input; ModbusResponse output; FTInterfaceStatus output; SerialIn input uint16; ResponseLength local; SerialOut output; LastModbusFunction local; MODBUS_TIMEOUT parameter; STREAMING_TIMEOUT parameter; Valid local
  function parseStreamingData:
    | function parseStreamingData %#codegen
    |     [GaugeCount, Gauge, SerialBuffer, SerialBufferEnd, GaugeStatus] = parseStreamingFTData(SerialIn, SerialBuffer, SerialBufferEnd);
    | end
  function clearSerialOut:
    | function clearSerialOut %#codegen
    |     SerialOut = zeros(256,1, 'uint16');
    | end
  function sendModbusCmd(Command):
    | function sendModbusCmd(Command) %#codegen
    |     
    |     % All ATI Digital F/T interface boards use Modbus address 10.
    |     % See ATI Digital F/T System Installation and Operation Manual
    |     % (Document #9620-05-Digital FT).
    |     ModbusAddress  = uint16(10); 
    |     ModbusFunction = Command(2);
    |     ModbusData     = Command(1+(2:Command(1)));
    |     ModbusPacket   = createModbusPacket(ModbusAddress, ModbusFunction, ModbusData);
    |     
    |     L = length(ModbusPacket);
    |     SerialOut(1)     = uint16(L);
    |     SerialOut(2:L+1) = ModbusPacket;
    |     
    |     % Expected response length
    |     ResponseLength = getModbusResponseLength(ModbusFunction, ModbusData);
    |     
    |     % Capture function
    |     LastModbusFunction = ModbusFunction;
    | end
  function sendStreamingCmd(Select):
    | function sendStreamingCmd(Select) %#codegen
    |     
    |     Function = uint16(70);
    |     if (Select==1)
    |         L = 2;
    |         Data = 85;
    |     else
    |         L = 16;
    |         Data = 85*ones(L-1,1,'uint16'); % JAMMING SEQUENCE
    |     end
    |     sendModbusCmd(uint16([L; Function; Data])) %#codegen
    | end
  function clearGauge:
    | function clearGauge %#codegen
    |     Gauge = zeros(6,8);
    |     GaugeCount = 0;
    |     %GaugeStatus = 0;
    |     GaugeStatus = zeros(8,1);
    | end
  function readModbusResponse:
    | function readModbusResponse %#codegen
    |     [Valid, SerialBuffer, SerialBufferEnd] = bufferModbusData(LastModbusFunction, ResponseLength, SerialIn, SerialBuffer, SerialBufferEnd);
    | end
  function validateModbusResponse:
    | function validateModbusResponse %#codegen
    |     Valid = false;
    |     ModbusResponse = zeros(256,1,'uint16');
    |     
    |     if (SerialBuffer(2) == LastModbusFunction) && (SerialBufferEnd == 3 + ResponseLength) ...
    |             || (SerialBuffer(2) == LastModbusFunction + 128) && (SerialBufferEnd == 5)
    |         
    |         Valid = checkModbusCRC(SerialBuffer(1:SerialBufferEnd));
    |         if Valid
    |             % Strip off the Modbus Address and CRC
    |             L = SerialBufferEnd-3;
    |             ModbusResponse(1) = uint16(L);
    |             ModbusResponse(1+(1:L)) = SerialBuffer(1+(1:L));
    |         end
    |     end
    | end
  function clearSerialBuffer:
    | function clearSerialBuffer %#codegen
    |     SerialBuffer = zeros(512,1,'uint16');
    |     SerialBufferEnd = uint16(0);
    | end
  function clearModbusResponse:
    | function clearModbusResponse %#codegen
    |     ModbusResponse(1) = uint16(0);
    |     ModbusStatus = 0;
    | end

== matlab function FTTest07/ComputeCalibratedTorques/ComputeCalibratedTorques ==
  data: Gauge input; FT output; Bias input; Cal input
function FT = fcn(Gauge, Bias, Cal)
    %#codegen
    FT = Cal.BasicMatrix * (Gauge - Bias);
    FT(1:3,:) = FT(1:3,:) / Cal.CountsPerForce;
    FT(4:6,:) = FT(4:6,:) / Cal.CountsPerTorque;
end
